simulink library "visionutilities"  (R2024b)
settings: Solver=ode45  StartTime=0.0  StopTime=10.0  RelTol=1e-3
values from neighbouring files (symbols this model uses):
  M = tform.T(1:D,1:D)    [bboxwarp.m]
  sz = size(cBlockSets,1)    [balanceBoxLabels.m]    (also in detectMSERFeatures.m = int32(imageSize); detectSURFFeatures.m = size(Iu8); estimateCameraParameters.m = size(allImagePoints))
undefined symbols (not defined in the file or in its folder): N
libraries: vipmisc x3
settings Model: Creator=The MathWorks, Inc.  LastModifiedBy=The MathWorks, Inc.
settings SolverCC: AlgebraicLoopSolver=TrustRegion  MaxZcPerStep=1
settings DataIOCC: LimitDataPoints=on  SaveFormat=Array  SignalLoggingSaveFormat=ModelDataLogs  ReturnWorkspaceOutputs=off
settings OptimizationCC: BlockReduction=off  BooleanDataType=off  ExpressionDepthLimit=2147483647  LifeSpan=inf
settings DebuggingCC: SaveWithParameterizedLinksMsg=none  UnderspecifiedInitializationDetection=Classic  MergeDetectMultiDrivingBlocksExec=none  SignalResolutionControl=TryResolveAllWithWarning  FcnCallInpInsideContextMsg=warning  UnconnectedInputMsg=warning  UnconnectedOutputMsg=warning  UnconnectedLineMsg=warning  StateNameClashWarn=warning  SFUnexpectedBacktrackingDiag=warning  SFNoUnconditionalDefaultTransitionDiag=warning  SFExecutionAtInitializationDiag=none  ArithmeticOperatorsInVariantConditions=warning
settings HardwareCC: ProdBitPerPointer=32  ProdBitPerSizeT=32  ProdBitPerPtrDiffT=32  ProdLargestAtomicFloat=None  ProdIntDivRoundTo=Undefined  ProdEndianess=Unspecified  ProdWordSize=32  ProdHWDeviceType=32-bit Generic  TargetUnknown=on
settings ModelReferenceCC: EnableRefExpFcnMdlSchedulingChecks=on  PropagateSignalLabelsOutOfModel=off
settings SFSimCC: SimUseLocalCustomCode=off  CustomCodeUndefinedFunction=UseInterfaceOnly
settings RTWCC: RTWUseLocalCustomCode=off  GPUComputeCapability=3.5  DLArmComputeVersion=19.05
settings CodeAppCC: StateflowObjectComments=on
settings GRTTargetCC: TargetLangStandard=C89/C90 (ANSI)  CombineOutputUpdateFcns=off  GRTInterface=on
settings ConfigComp: CovMetricSettings=dw  CovSaveCumulativeToWorkspaceVar=on  CovSaveSingleToWorkspaceVar=on  CovExternalEMLEnable=off

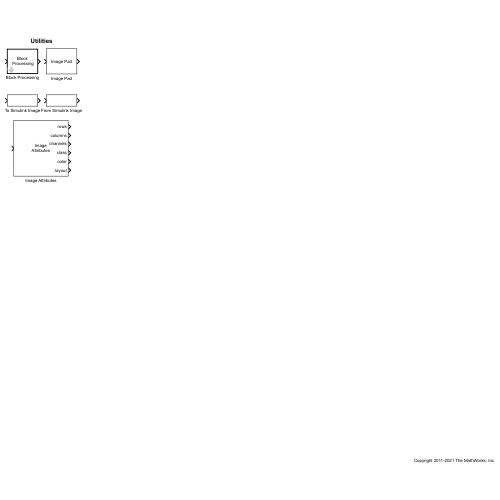
[thumbnail: Simulink's stored preview of the top-level diagram]
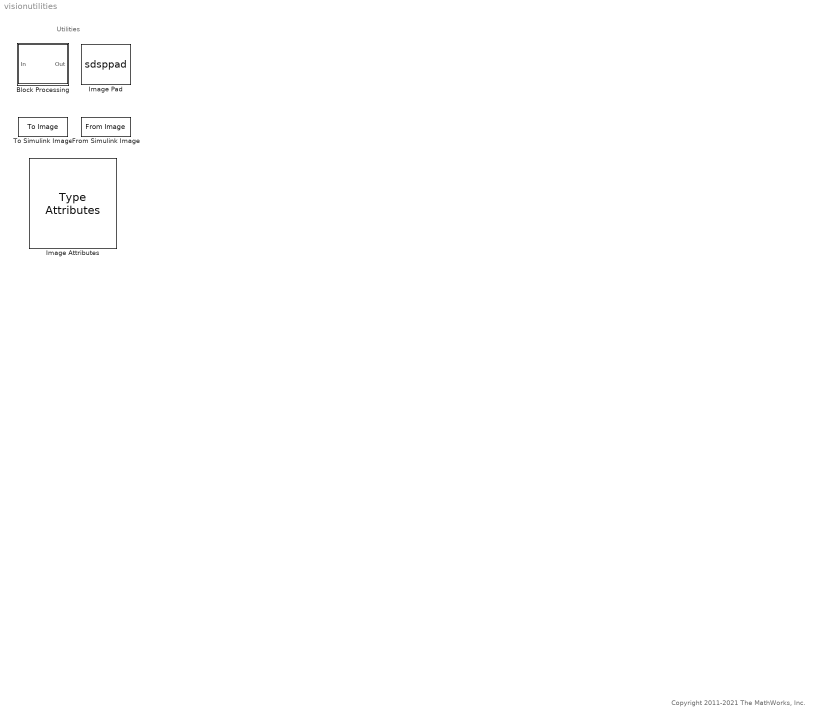
== system visionutilities ==
  note: Utilities
  note: Copyright 2011-2021 The MathWorks, Inc.
  Block Processing : Subsystem  TreatAsAtomicUnit=on  mask(Block Processing){NumI=1, ParamPort=off, NumO=1, Blocksize={[8 8]}, Overlapsize={[0 0]}, Traverse=Row-wise}
      mask prompts: NumI "vision:masks:NumberOfInputs"; ParamPort "vision:masks:AddPortToSupplySubsystemParam"; NumO "vision:masks:NumberOfOutputs"; Blocksize "vision:masks:BlockSize"; Overlapsize "vision:masks:OverlapSize"; Traverse "vision:masks:TraverseOrder"
      mask help: vision:masks:BlockProcessingDescription
      mask init:
      | errmsg = vipblkblockproc(gcbh, NumI, NumO, Blocksize, Overlapsize, Traverse, ParamPort);
      | error(errmsg);
      settings: CopyFcn=set_param(gcb,'LinkStatus','none');
      mask Help: helpview('vision','BlockProcessingSimulink');
      mask TypeOptions Traverse: vision:masks:Rowwise | vision:masks:Columnwise
      mask DialogControl NumI Prompt: Number of inputs:
      mask DialogControl ParamPort Prompt: Add port to supply subsystem parameters
      mask DialogControl NumO Prompt: Number of outputs:
      mask DialogControl Blocksize Prompt: Block size:
      mask DialogControl Overlapsize Prompt: Overlap size:
      mask DialogControl Traverse Prompt: Traverse order:
      mask DialogControl subsystemGrpBox Prompt: vision:masks:Subsystem
      mask DialogControl subsystemText Prompt: vision:masks:ClickTheOpenSubsystemButton
      mask DialogControl openSubsystem Prompt: vision:masks:OpenSubsystem
      mask DialogControl openSubsystem Callback: Opensubsystem(gcbh)
      mask Display:
      | disp('Block\n Processing');
      | 
      | if ((NumI == 1) && ParamPort)
      |     port_label('input', 1, 'I');
      | end
      | 
      | if (NumI > 1)
      |     for (i = 1:NumI)
      |         port_label('input', i, ['I' int2str(i)]);
      |     end
      | end
      | 
      | if (ParamPort)
      |     port_label('input', NumI+1, 'P');
      | end
  From Simulink Image : FromImage
  Image Attributes : TypeAttributes  mask(ImageAttributes){}
      mask help: SimulinkBlocks:ImageBlocks:ImageAttributesDescription
      mask Help: helpview('vision','block_imageattributes');
      mask Display:
      | disp('Image\nAttributes');
      | port_label('output', 1, 'rows');
      | port_label('output', 2, 'columns');
      | port_label('output', 3, 'channels');
      | port_label('output', 4, 'class');
      | port_label('output', 5, 'color');
      | port_label('output', 6, 'layout');
  Image Pad : S-Function  FunctionName=sdsppad  Parameters=method,valSrc,value,spec,outColsMode,rowDirection,rowSize,outColSize,outRowsMode,colDirection,colSize,outRowSize,trunc_flag,0,0,0,0,0,0,0,2  SFunctionDeploymentMode=off  EnableBusSupport=on  mask(Image Pad){method=Constant, valSrc=Specify via dialog, value=0, spec=Pad size, rowDirection=Both left and right, outRowsMode=User-specified, rowSize=2, outColSize=10, colDirection=Both top and bottom, outColsMode=User-specified, colSize=[2 3], outRowSize=12, trunc_flag=None}
      mask prompts: method "vision:masks:Method"; valSrc "vision:masks:PadValueSource"; value "vision:masks:PadValue"; spec "vision:masks:Specify"; rowDirection "vision:masks:AddColumnsTo"; outRowsMode "vision:masks:OutputColumnMode"; rowSize "vision:masks:NumberOfAddedColumns"; outColSize "vision:masks:NumberOfOutputColumns"; colDirection "vision:masks:AddRowsTo"; outColsMode "vision:masks:OutputRowMode"; colSize "vision:masks:NumberOfAddedRows"; outRowSize "vision:masks:NumberOfOutputRows"; trunc_flag "vision:masks:ActionWhenTruncationOccurs"
      mask help: vision:masks:ImagePadDescription
      mask init:
      | ports = vipblk2dpad('icon');
      mask Help: eval('visionblockhelp');
      mask TypeOptions method: vision:masks:Constant | vision:masks:Replicate | vision:masks:Symmetric | vision:masks:Circular
      mask Callback method: vipblk2dpad
      mask TypeOptions valSrc: vision:masks:SpecifyViaDialog | vision:masks:InputPort
      mask Callback valSrc: vipblk2dpad
      mask TypeOptions spec: vision:masks:PadSize | vision:masks:OutputSizeValue
      mask Callback spec: vipblk2dpad
      mask TypeOptions rowDirection: vision:masks:Left | vision:masks:Right | vision:masks:BothLeftAndRight | vision:masks:NoPadding
      mask Callback rowDirection: vipblk2dpad
      mask TypeOptions outRowsMode: vision:masks:Userspecified | vision:masks:NextPowerOfTwo
      mask Callback outRowsMode: vipblk2dpad
      mask TypeOptions colDirection: vision:masks:Top | vision:masks:Bottom | vision:masks:BothTopAndBottom | vision:masks:NoPadding
      mask Callback colDirection: vipblk2dpad
      mask TypeOptions outColsMode: vision:masks:Userspecified | vision:masks:NextPowerOfTwo
      mask Callback outColsMode: vipblk2dpad
      mask TypeOptions trunc_flag: vision:masks:None | vision:masks:Warning | vision:masks:Error
      mask DialogControl method Prompt: Method:
      mask DialogControl valSrc Prompt: Pad value source:
      mask DialogControl value Prompt: Pad value:
      mask DialogControl spec Prompt: Specify:
      mask DialogControl rowDirection Prompt: Add columns to:
      mask DialogControl outRowsMode Prompt: Output column mode:
      mask DialogControl rowSize Prompt: Number of added columns:
      mask DialogControl outColSize Prompt: Number of output columns:
      mask DialogControl colDirection Prompt: Add rows to:
      mask DialogControl outColsMode Prompt: Output row mode:
      mask DialogControl colSize Prompt: Number of added rows:
      mask DialogControl outRowSize Prompt: Number of output rows:
      mask DialogControl trunc_flag Prompt: Action when truncation occurs:
      mask Display:
      | disp('Image Pad');
      | port_label('input',ports.port1, ports.txt1);
      | port_label('input',ports.port2, ports.txt2);
      | port_label('output',ports.port3, ports.txt3);
  To Simulink Image : ToImage

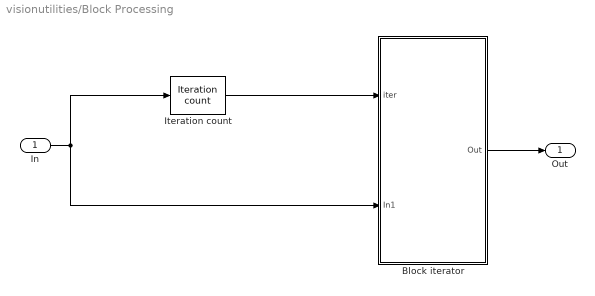
== system visionutilities/Block Processing ==
  In : Inport
  Block iterator : Subsystem
      settings: CopyFcn=set_param(gcb,'ReferenceBlock','');
  Iteration count : vipmisc/Iteration count  NumI=NumI  blksize=Blocksize  ovlpsize=Overlapsize
  Out : Outport  VectorParamsAs1DForOutWhenUnconnected=off
  wires:
  Block iterator/1(Out) -> Out/1
  In/1 -> Block iterator/2(In1), Iteration count/1
  Iteration count/1 -> Block iterator/1(iter)

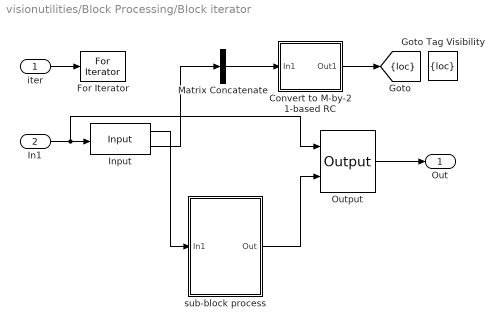
== system visionutilities/Block Processing/Block iterator ==
  iter : Inport
  In1 : Inport  Port=2
  Convert to M-by-2 1-based RC : Subsystem
  For Iterator : ForIterator  IterationSource=external  IterationLimit=(sz(1)/M)*(sz(2)/N)  ShowIterationPort=off  IndexMode=Zero-based  IterationVariableDataType=double
  Goto Tag Visibility : GotoTagVisibility  GotoTag=loc
  Input : vipmisc/Input  Blocksize=Blocksize{1}  Overlapsize=Overlapsize{1}  tverse=Row-wise
  Matrix Concatenate : Concatenate  NumInputs=1  Mode=Multidimensional array  ConcatenateDimension=2
  Output : vipmisc/Output  Blocksize=Blocksize{1}  Overlapsize=Overlapsize{1}  tverse=Row-wise
  sub-block process : Subsystem
  Out : Outport  VectorParamsAs1DForOutWhenUnconnected=off
  tag scope: loc=scoped
  wires:
  sub-block process/1(Out) -> Output/2
  Output/1 -> Out/1
  In1/1 -> Output/1, Input/1
  iter/1 -> For Iterator/1
  Input/1 -> sub-block process/1(In1)
  Input/2 -> Matrix Concatenate/1
  Matrix Concatenate/1 -> Convert to M-by-2 1-based RC/1(In1)
  Convert to M-by-2 1-based RC/1(Out1) -> [loc]

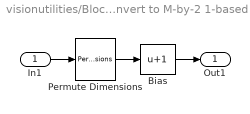
== system visionutilities/Block Processing/Block iterator/Convert to M-by-2 1-based RC ==
  In1 : Inport
  Bias : Bias  Bias=1  SaturateOnIntegerOverflow=off
  Permute Dimensions : PermuteDimensions
  Out1 : Outport  VectorParamsAs1DForOutWhenUnconnected=off
  wires:
  Permute Dimensions/1 -> Bias/1
  Bias/1 -> Out1/1
  In1/1 -> Permute Dimensions/1

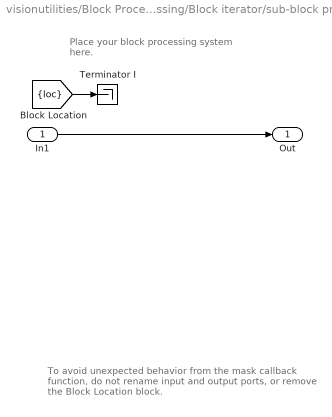
== system visionutilities/Block Processing/Block iterator/sub-block process ==
  note: Place your block
      | processing system here.
  note: To avoid unexpected behavior from the mask
      | callback function, do not rename input and output ports,
      | or remove the Block Location block.
  In1 : Inport
  Terminator I : Terminator
  Out : Outport  VectorParamsAs1DForOutWhenUnconnected=off
  wires:
  In1/1 -> Out/1
  [loc] -> Terminator I/1
